simulink model "rtwdemo_requirements"  (Simulink 6.0)
settings: Solver=FixedStepDiscrete  SolverMode=SingleTasking  StartTime=0.0  StopTime=0.1  FixedStep=0.001  RelTol=1e-3
PreLoadFcn:
  | timestamps = 0.1:0.2:49.8;
  | t=[0, timestamps, timestamps, 50];
  | t = 0.01 + sort(t)';
  | u = [zeros(1,25);zeros(1,25);zeros(1,25);zeros(1,25);zeros(1,25);zeros(1,25);ones(1,25);ones(1,25);zeros(1,25);zeros(1,25);ones(1,25);ones(1,25);ones(1,25);ones(1,25);ones(1,25);ones(1,25);ones(1,25);ones(1,25);ones(1,25);ones(1,25)];
  | u = u(:);
  | rebound1_input = [t,u];
PostLoadFcn:
  | INC=uint8(1);LIMIT=uint8(16);RESET=uint8(0);K=int32(2);
undefined symbols (not defined in the file or in its folder): sigbuilder_block
libraries: rtwdemowidgets x1
settings Model: CovMetricSettings=d  Creator=The MathWorks Inc.  LastModifiedBy=batserve  ParamWorkspaceSource=ReferencedWorkspace  ExtModeTrigMode=oneshot  ExtModeArmWhenConnect=off  ExtModeAutoUpdateStatusClock=off
settings DataIOCC: LimitDataPoints=off  SaveFormat=StructureWithTime  SaveOutput=off  SaveTime=off  SignalLoggingName=sigsOut
settings OptimizationCC: InlineParams=on  EnforceIntegerDowncast=off  StateBitsets=on  DataBitsets=on  UseTempVars=on  ZeroExternalMemoryAtStartup=off  ZeroInternalMemoryAtStartup=off  InitFltsAndDblsToZero=off  NoFixptDivByZeroProtection=on  OptimizeModelRefInitCode=on  LifeSpan=1
settings DebuggingCC: CheckExecutionContextPreStartOutputMsg=on  CheckExecutionContextRuntimeOutputMsg=on  SolverPrmCheckMsg=none  IntegerOverflowMsg=none
settings ModelReferenceCC: UpdateModelReferenceTargets=IfOutOfDate
settings RTWCC: SystemTargetFile=ert.tlc  TLCOptions=-p0 -aWarnNonSaturatedBlocks=0  TemplateMakefile=ert_default_tmf  GenerateReport=on  RTWVerbose=off  ProcessScript=ert_make_rtw_hook  IncludeHyperlinkInReport=on  LaunchReport=on
settings CodeAppCC: ForceParamTrailComments=on  IgnoreCustomStorageClasses=off  SimulinkDataObjDesc=on  PrefixModelToSubsysFcnNames=off  CustomSymbolStr=$N$M  InsertBlockDesc=on  ReqsInCode=on
settings ERTTargetCC: TargetFcnLib=ansi_tfl_tmw.mat  GenFloatMathFcnCalls=ANSI_C  GenerateSampleERTMain=on  IncludeMdlTerminateFcn=off  SupportNonFinite=off  SupportContinuousTime=on  SupportNonInlinedSFcns=on  InlinedParameterPlacement=NonHierarchical  RootIOFormat=Individual Arguments  ERTCustomFileTemplate=example_file_process.tlc  InitialValueSource=Model

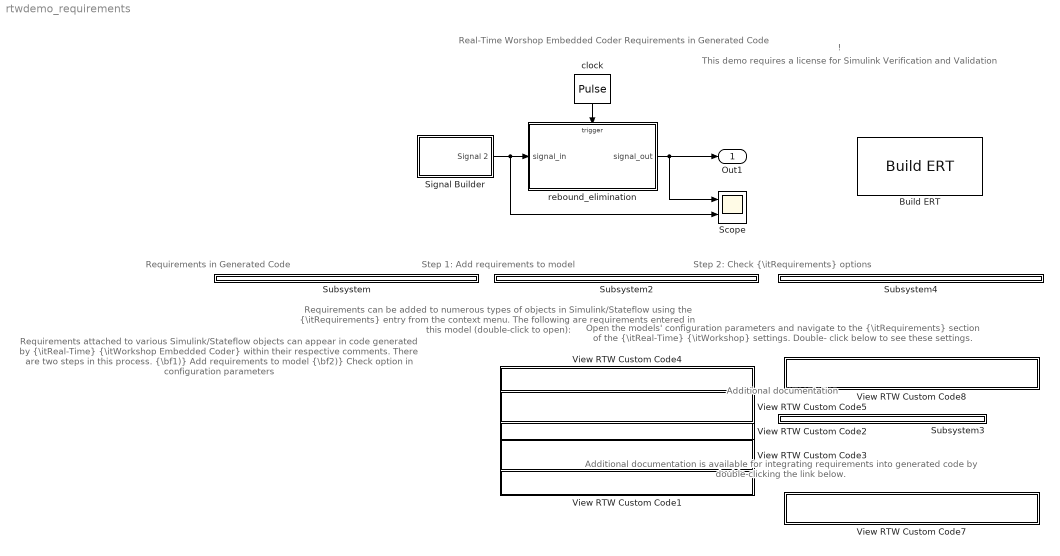
== system rtwdemo_requirements ==
  note: Real-Time Worshop Embedded Coder
      | Requirements in Generated Code
  note: This demo requires a license for
      | Simulink Verification and Validation
  note: !
  note: Requirements attached to various
      | Simulink/Stateflow objects can appear
      | in code generated by {\itReal-Time}
      | {\itWorkshop Embedded Coder} within their
      | respective comments.  There are
      | two steps in this process.
      |
      | {\bf1)} Add requirements to model
      | {\bf2)} Check option in configuration parameters
  note: Requirements in Generated Code
  note: Requirements can be added to numerous types
      | of objects in Simulink/Stateflow using the
      | {\itRequirements} entry from the context menu.
      | The following are requirements entered in
      | this model (double-click to open):
  note: Step 1: Add requirements to model
  note: Open the models' configuration parameters and
      | navigate to the {\itRequirements} section of the
      | {\itReal-Time} {\itWorkshop} settings.  Double-
      | click below to see these settings.
  note: Step 2: Check {\itRequirements} options
  note: Additional documentation
  note: Additional documentation is available
      | for integrating requirements into
      | generated code by double-clicking the
      | link below.
  Build ERT : rtwdemowidgets/Build ERT  attrib_overrides={}
  Scope : Scope  NumInputPorts=2
      settings: YMin=0~0  YMax=1~1
  Signal Builder : Subsystem  Tag=STV Subsys  RequirementInfo={'other' '' '' 'true' '111' '' }  LoadFcn=sigbuilder_block('load');  StartFcn=sigbuilder_block('start');  StopFcn=sigbuilder_block('stop');  ClipboardFcn=sigbuilder_block('clipboard');  PropExecContextAcrossSSBoundary=on  mask(Sigbuilder block){}
      mask help: Sigbuilder GUI
      mask init:
      | if ~strcmp(get_param(bdroot(gcbh),'SimulationStatus'),'stopped') tuvar = sigbuilder_block('maskInit'); end
      settings: CopyFcn=sigbuilder_block('copy');  DeleteFcn=sigbuilder_block('delete');  ModelCloseFcn=sigbuilder_block('modelClose');  PreSaveFcn=sigbuilder_block('preSave');  NameChangeFcn=sigbuilder_block('namechange');  OpenFcn=sigbuilder_block('open',[72.75 51.75 599.25 399.75 ]);  CloseFcn=sigbuilder_block('close');
      mask Display: plot(0,0,100,100,[10,10,40,40,10],[80,20,20,80,80],[40,10],[50,50], [40,27,10],[65,72,56],[40,25,25,10],[28,28,43,43]);
  Subsystem : Subsystem  PropExecContextAcrossSSBoundary=on
  Subsystem2 : Subsystem  PropExecContextAcrossSSBoundary=on
  Subsystem3 : Subsystem  PropExecContextAcrossSSBoundary=on
  Subsystem4 : Subsystem  PropExecContextAcrossSSBoundary=on
  View RTW Custom Code1 : Subsystem  PropExecContextAcrossSSBoundary=on
      mask init:
      | pos    = get_param(gcb, 'Position');
      | width  = pos(3) - pos(1);
      | height = pos(4) - pos(2);
      | 
      | 
      | % Compute arrow coordinates
      | arrowW = width  / 20;
      | arrowH = height / 2.5;
      | arrowX = width  / 50;
      | arrowY = height / 3;
      | arrowXvec = [arrowX, arrowX, arrowX + arrowW];
      | arrowYvec = [arrowY, arrowY + arrowH, arrowY + arrowH / 2];
      | 
      | % Compute text position
      | textXbuff = width / 30;
      | textX  = arrowX + arrowW + textXbuff;
      | textY  = height / 2;
      settings: OpenFcn=|
      | clockblock='rtwdemo_requirements/clock';
      | sigbblock='rtwdemo_requirements/Signal Builder';
      | hilite_system(sigbblock,'none');
      | hilite_system(clockblock,'none');
      | func=find(sfroot,'-isa','Stateflow.Function','-and','Tag','req_function');
      | sf('Open',func.id);
      | rmi('edit',func.id);
      mask Display:
      | patch(arrowXvec, arrowYvec);
      | text(textX, textY, 'Stateflow Graphical Function');
  View RTW Custom Code2 : Subsystem  PropExecContextAcrossSSBoundary=on
      mask init: same as rtwdemo_requirements/View RTW Custom Code1
      settings: OpenFcn=|
      | clockblock='rtwdemo_requirements/clock';
      | sigbblock='rtwdemo_requirements/Signal Builder';
      | hilite_system(sigbblock,'none');
      | hilite_system(clockblock,'none');
      | trans=find(sfroot,'-isa','Stateflow.Transition','-and','Tag','req_trans');
      | sf('Open',trans.id);
      | rmi('edit',trans.id);
      mask Display:
      | patch(arrowXvec, arrowYvec);
      | text(textX, textY, 'Stateflow State');
  View RTW Custom Code3 : Subsystem  PropExecContextAcrossSSBoundary=on
      mask init: same as rtwdemo_requirements/View RTW Custom Code1
      settings: OpenFcn=|
      | clockblock='rtwdemo_requirements/clock';
      | sigbblock='rtwdemo_requirements/Signal Builder';
      | hilite_system(sigbblock,'none');
      | hilite_system(clockblock,'none');
      | trans=find(sfroot,'-isa','Stateflow.Transition','-and','Tag','req_trans');
      | sf('Open',trans.id);
      | rmi('edit',trans.id);
      mask Display:
      | patch(arrowXvec, arrowYvec);
      | text(textX, textY, 'Stateflow Transition');
  View RTW Custom Code4 : Subsystem  PropExecContextAcrossSSBoundary=on
      mask init: same as rtwdemo_requirements/View RTW Custom Code1
      settings: OpenFcn=|
      | clockblock='rtwdemo_requirements/clock';
      | sigbblock='rtwdemo_requirements/Signal Builder';
      | clockblockh=get_param(clockblock,'handle');
      | hilite_system(sigbblock,'none');
      | hilite_system(clockblockh);
      | rmi('edit',clockblockh);
      mask Display:
      | patch(arrowXvec, arrowYvec);
      | text(textX, textY, 'Simulink Block');
  View RTW Custom Code5 : Subsystem  PropExecContextAcrossSSBoundary=on
      mask init: same as rtwdemo_requirements/View RTW Custom Code1
      settings: OpenFcn=|
      | sigbblock='rtwdemo_requirements/Signal Builder';
      | clockblock='rtwdemo_requirements/clock';
      | hilite_system(clockblock,'none');
      | hilite_system(sigbblock);
      | open_system(sigbblock);
      mask Display:
      | patch(arrowXvec, arrowYvec);
      | text(textX, textY, 'Simulink Signal Builder');
  View RTW Custom Code7 : Subsystem  PropExecContextAcrossSSBoundary=on
      mask init: same as rtwdemo_requirements/View RTW Custom Code1
      settings: OpenFcn=helpview([docroot '/mapfiles/slvnv.map'], 'managing_modeling_requirements')
      mask Display:
      | patch(arrowXvec, arrowYvec);
      | text(textX, textY, 'Requirements Documentation');
  View RTW Custom Code8 : Subsystem  PropExecContextAcrossSSBoundary=on
      mask init: same as rtwdemo_requirements/View RTW Custom Code1
      settings: OpenFcn=|
      | model = bdroot;
      | slCfgPrmDlg(model,'Open');
      | slCfgPrmDlg(bdroot,'TurnToPage','Comments');
      mask Display:
      | patch(arrowXvec, arrowYvec);
      | text(textX, textY, 'Open Requirements Settings');
  clock : DiscretePulseGenerator  RequirementInfo={'other' 'rtwdemo_requirements_doc.html' 'Requirement 5' 'true' 'Clock period shall be consistent with chirp tolerance' '' }  Orientation=down  PulseType=Time based  Period=0.002  PulseWidth=50
  rebound_elimination : Stateflow chart  PropExecContextAcrossSSBoundary=on
  Out1 : Outport
  wires:
  Signal Builder/1(Signal 2) -> Scope/2, rebound_elimination/1(signal_in)
  rebound_elimination/1(signal_out) -> Scope/1, Out1/1
  clock/1 -> rebound_elimination/Trigger

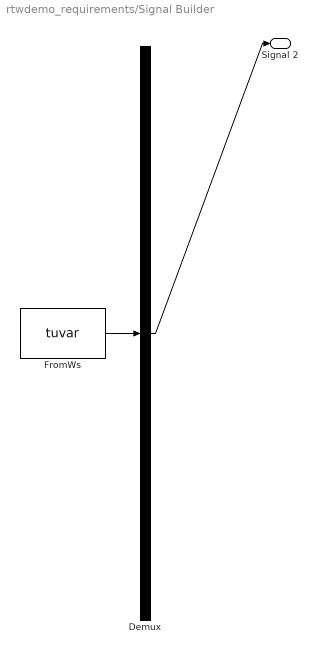
== system rtwdemo_requirements/Signal Builder ==
  Demux : Demux  Tag=STV Demux  Outputs=1
  FromWs : FromWorkspace  Tag=STV FromWs  VariableName=tuvar  SampleTime=0  SigBuilderData=DataTag0  VnvData=DataTag1
      SigBuilderData=|
      | channels.label = 'Signal 2'
      | channels.allXData = {[0 0.0011 0.0011 0.0031 0.0031 0.0051 0.0051 0.0071 0.0071 0.0091 0.0091 0.0111 0.0111 0.0131 0.0131 0.0151 0.0151 0.0171 0.0171 0.0191 0.0191 0.0211 0.0211 0.0231 0.0231 0.0251 0.0251 0.0271 0.0271 0.0291 0.0291 0.0311 0.0311 0.0331 0.0331 0.0351 0.0351 0.0371 0.0371 0.0391 0.0391 0.0411 0.0411 0.0431 0.0431 0.0451 0.0451 0.0471 0.0471 0.0491 0.0491 0.0511 0.0511 0.0531 0.0531 0.0551 0.0551 0.0571 0.0571 0.0591 0.0591 0.0611 0.0611 0.0631 0.0631 0.0651 0.0651 0.0671 0.0671 0.0691 0.0691 0.0711 0.0711 0.0731 0.0731 0.0751 0.0751 0.0771 0.0771 0.0791 0.0791 0.0811 0.0811 0.0831 0.0831 0.0851 0.0851 0.0871 0.0871 0.0891 0.0891 0.0911 0.0911 0.0931 0.0931 0.0951 0.0951 0.0971 0.0971 0.0991 0.0991 0.1], [0 0.0011 0.0011 0.0031 0.0031 0.0051 0.0051 0.0071 0.0071 0.0091 0.0091 0.0111 0.0111 0.0131 0.0131 0.0151 0.0151 0.0171 0.0171 0.0191 0.0191 0.0211 0.0211 0.0231 0.0231 0.0251 0.0251 0.0271 0.0271 0.0291 0.0291 0.0311 0.0311 0.0331 0.0331 0.0351 0.0351 0.0371 0.0371 0.0391 0.0391 0.0411 0.0411 0.0431 0.0431 0.0451 0.0451 0.0471 0.0471 0.0491 0.0491 0.0511 0.0511 0.0531 0.0531 0.0551 0.0551 0.0571 0.0571 0.0591 0.0591 0.0611 0.0611 0.0631 0.0631 0.0651 0.0651 0.0671 0.0671 0.0691 0.0691 0.0711 0.0711 0.0731 0.0731 0.0751 0.0751 0.0771 0.0771 0.0791 0.0791 0.0811 0.0811 0.0831 0.0831 0.0851 0.0851 0.0871 0.0871 0.0891 0.0891 0.0911 0.0911 0.0931 0.0931 0.0951 0.0951 0.0971 0.0971 0.0991 0.0991 0.1]}
      | channels.allYData = {[0 0 0 0 0 0 1 1 0 0 1 1 1 1 1 1 1 1 1 1 0 0 0 0 0 0 1 1 0 0 1 1 1 1 1 1 1 1 1 1 0 0 0 0 0 0 1 1 0 0 1 1 1 1 1 1 1 1 1 1 0 0 0 0 0 0 1 1 0 0 1 1 1 1 1 1 1 1 1 1 0 0 0 0 0 0 1 1 0 0 1 1 1 1 1 1 1 1 1 1 0 0], [1 1 1 1 1 1 1 1 1 1 0 0 1 1 0 0 0 0 0 0 1 1 1 1 1 1 1 1 1 1 0 0 1 1 0 0 0 0 0 0 1 1 1 1 1 1 1 1 1 1 0 0 1 1 0 0 0 0 0 0 1 1 1 1 1 1 1 1 1 1 0 0 1 1 0 0 0 0 0 0 1 1 1 1 1 1 1 1 1 1 0 0 1 1 0 0 0 0 0 0 1 1]}
      | dataSet(1).timeRange = [0 0.1]
      | dataSet(1).name = 'Leading Chirp'
      | dataSet(2).timeRange = [0 0.1]
      | dataSet(2).name = 'Lagging Chirp'
  Signal 2 : Outport  Tag=STV Outport
  wires:
  FromWs/1 -> Demux/1
  Demux/1 -> Signal 2/1

== system rtwdemo_requirements/Subsystem ==

== system rtwdemo_requirements/Subsystem2 ==

== system rtwdemo_requirements/Subsystem3 ==

== system rtwdemo_requirements/Subsystem4 ==

== system rtwdemo_requirements/View RTW Custom Code1 ==

== system rtwdemo_requirements/View RTW Custom Code2 ==

== system rtwdemo_requirements/View RTW Custom Code3 ==

== system rtwdemo_requirements/View RTW Custom Code4 ==

== system rtwdemo_requirements/View RTW Custom Code5 ==

== system rtwdemo_requirements/View RTW Custom Code7 ==

== system rtwdemo_requirements/View RTW Custom Code8 ==

== stateflow chart rebound_elimination ==
  state rebound_state
    during:
    signal_out = rebound_fcn(previous_input, previous_output, signal_in);
    previous_input = signal_in;
    previous_output = signal_out;
  state result=rebound_fcn(prev_in, prev_out, curr_in) [function]
    (default) -> (junction 5)
    (junction 5) -> (junction 6) : [prev_in == curr_in]
        | {result = curr_in;}
    (junction 5) -> (junction 7)
    (junction 7) -> (junction 8) : {result = prev_out;}
  (default) -> rebound_state : {
      | previous_input = 0;
      | previous_output = 0;
      | }
  data: prev_in function_input double size=1; prev_out function_input double size=1; curr_in function_input double size=1; result function_output double size=1; signal_in input inherited; signal_out output double size=1; previous_input local double size=1; previous_output local double size=1
  events: event input RISING_EDGE_EVENT
